simulink model "robotarm_individual"  (R2018b)
settings: Solver=FixedStepAuto  StartTime=0.0  StopTime=options.T_train-options.dt  RelTol=1e-3  AbsTol=1e-6
undefined symbols (not defined in the file or in its folder): options
libraries: neural x132, simulink x4
(part 2 of 6)

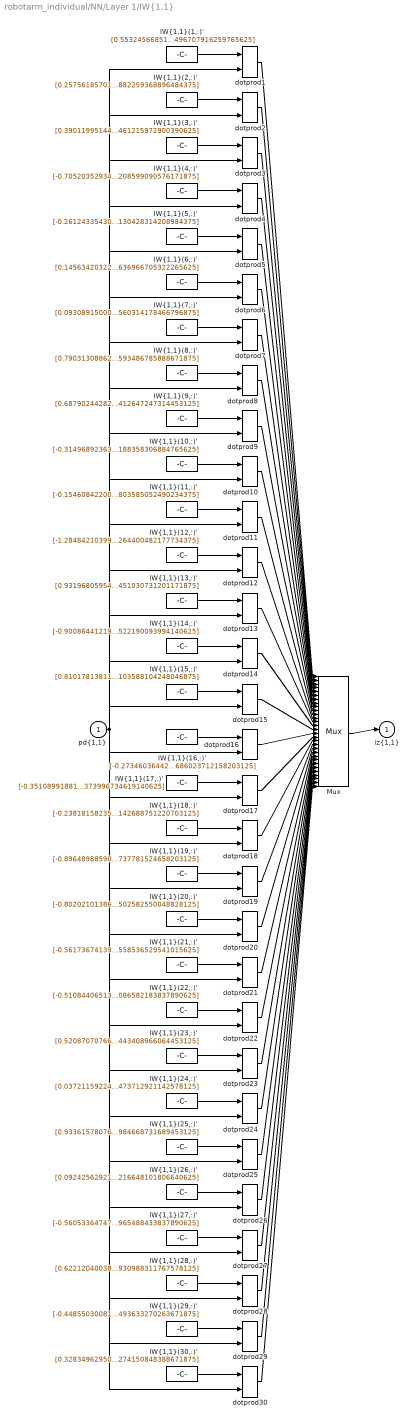
== system robotarm_individual/NN/Layer 1/IW{1,1} ==
  "pd{1,1}" : Inport  PortDimensions=10
      mask Display: e = 0.06;c1 = [120 230 180]/255;c2 = ([120 230 180]+0)/(256+128);c3 = ([120 230 180]+128)/(256+128);patch([0 1 1 0],[0 0 1 1],c1);patch([0 1 1 1-e 1-e 0+e],[0 0 1 1-e 0+e 0+e],c2);patch([0 0 1 1-e 0+e 0+e],[0 1 1 1-e 1-e 0+e],c3);plot([0 1 1 0 0],[0 0 1 1 0]);
  "IW{1,1}(1,:)'" : Constant  Value=[0.5532456685171613930407374937203712761402130126953125;-0.378274693650503757158531925597344525158405303955078125;0.56914966942954603457138773592305369675159454345703125;-0.50553199151917294074110031942836940288543701171875;0.658232888932551052363351118401624262332916259765625;-0.94884153385445257899988291683257557451725006103515625;0.473460329120412637404768929627607576549053192138671875;-0.343214399203028375229251878408831544220447540283203125;-0.86431174897959639480404803180135786533355712890625;0.589926606124411279097330407239496707916259765625]
      mask Display: e = 0.06;c1 = [120 150 230]/255;c2 = ([120 150 230]+0)/383;c3 = ([120 150 230]+128)/383;patch([0 1 1 0],[0 0 1 1],c1);patch([0 1 1 1-e 1-e 0+e],[0 0 1 1-e 0+e 0+e],c2);patch([0 0 1 1-e 0+e 0+e],[0 1 1 1-e 1-e 0+e],c3);plot([0 1 1 0 0],[0 0 1 1 0]);disp('Weights');
  "IW{1,1}(10,:)'" : Constant  Value=[-0.31496892363713457907437032190500758588314056396484375;0.08016139377854337999540490500294254161417484283447265625;-0.61410989189934184206975942288408987224102020263671875;0.83386729739820009132955647146445699036121368408203125;0.57799131071100695589137785646016709506511688232421875;-0.6262339995467105513426986362901516258716583251953125;-0.7518840900690875184153583177248947322368621826171875;-0.26218799647532831098573069539270363748073577880859375;0.8278812331514815436861454145400784909725189208984375;0.08425980137559320459761380561758414842188358306884765625]
      mask Display: e = 0.06;c1 = [120 150 230]/255;c2 = ([120 150 230]+0)/383;c3 = ([120 150 230]+128)/383;patch([0 1 1 0],[0 0 1 1],c1);patch([0 1 1 1-e 1-e 0+e],[0 0 1 1-e 0+e 0+e],c2);patch([0 0 1 1-e 0+e 0+e],[0 1 1 1-e 1-e 0+e],c3);plot([0 1 1 0 0],[0 0 1 1 0]);disp('Weights');
  "IW{1,1}(11,:)'" : Constant  Value=[-0.154608422005096890483599736398900859057903289794921875;0.68411476946963423184655539444065652787685394287109375;1.2591100033743873876090901831048540771007537841796875;0.1916528314192149640149409606237895786762237548828125;0.73897937867888419116724207924562506377696990966796875;-0.462187568499372092301058501107036136090755462646484375;-0.6040747226094336230772796625387854874134063720703125;0.36621315421464040174015508455340750515460968017578125;-0.372145694478708488617257899022661149501800537109375;0.78331781670854760957212192806764505803585052490234375]
      mask Display: e = 0.06;c1 = [120 150 230]/255;c2 = ([120 150 230]+0)/383;c3 = ([120 150 230]+128)/383;patch([0 1 1 0],[0 0 1 1],c1);patch([0 1 1 1-e 1-e 0+e],[0 0 1 1-e 0+e 0+e],c2);patch([0 0 1 1-e 0+e 0+e],[0 1 1 1-e 1-e 0+e],c3);plot([0 1 1 0 0],[0 0 1 1 0]);disp('Weights');
  "IW{1,1}(12,:)'" : Constant  Value=[-1.28484210399403142588425907888449728488922119140625;0.22635365405415874828776168214972130954265594482421875;0.1816503187597983959289393851577187888324260711669921875;-0.1064881354629866605510102317566634155809879302978515625;-1.0462119922659776083406768520944751799106597900390625;0.5159786559938523975432644874672405421733856201171875;-0.8176738284437050641173527765204198658466339111328125;0.55055084348684513173566301702521741390228271484375;0.7383955129630279667907188922981731593608856201171875;0.19266224517703045560068630948080681264400482177734375]
      mask Display: e = 0.06;c1 = [120 150 230]/255;c2 = ([120 150 230]+0)/383;c3 = ([120 150 230]+128)/383;patch([0 1 1 0],[0 0 1 1],c1);patch([0 1 1 1-e 1-e 0+e],[0 0 1 1-e 0+e 0+e],c2);patch([0 0 1 1-e 0+e 0+e],[0 1 1 1-e 1-e 0+e],c3);plot([0 1 1 0 0],[0 0 1 1 0]);disp('Weights');
  "IW{1,1}(13,:)'" : Constant  Value=[0.93196805954806338778695362634607590734958648681640625;-0.3434030090779085497842970653437077999114990234375;0.26082198307258275260522850658162496984004974365234375;0.96324277405090830139755553318536840379238128662109375;-0.0628666554734025606610003933383268304169178009033203125;0.1961376834922242962111482711407006718218326568603515625;0.426206572939244632269861767781549133360385894775390625;-0.09830317045506797857257197392755188047885894775390625;-0.56255042861082971139552455497323535382747650146484375;-0.9320516091341672915149274558643810451030731201171875]
      mask Display: e = 0.06;c1 = [120 150 230]/255;c2 = ([120 150 230]+0)/383;c3 = ([120 150 230]+128)/383;patch([0 1 1 0],[0 0 1 1],c1);patch([0 1 1 1-e 1-e 0+e],[0 0 1 1-e 0+e 0+e],c2);patch([0 0 1 1-e 0+e 0+e],[0 1 1 1-e 1-e 0+e],c3);plot([0 1 1 0 0],[0 0 1 1 0]);disp('Weights');
  "IW{1,1}(14,:)'" : Constant  Value=[-0.9008644121983826469346468002186156809329986572265625;0.313446134367460327307952638875576667487621307373046875;0.96742102718049050036341895975056104362010955810546875;0.60793812066105668012738760808133520185947418212890625;-0.66596089840168570805900571940583176910877227783203125;0.184208381037875235097800441508297808468341827392578125;1.04809193563155833572864139568991959095001220703125;0.1271048703670402957310869851426105014979839324951171875;0.162963867020818276021287829280481673777103424072265625;0.14456201261527967805164962555863894522190093994140625]
      mask Display: e = 0.06;c1 = [120 150 230]/255;c2 = ([120 150 230]+0)/383;c3 = ([120 150 230]+128)/383;patch([0 1 1 0],[0 0 1 1],c1);patch([0 1 1 1-e 1-e 0+e],[0 0 1 1-e 0+e 0+e],c2);patch([0 0 1 1-e 0+e 0+e],[0 1 1 1-e 1-e 0+e],c3);plot([0 1 1 0 0],[0 0 1 1 0]);disp('Weights');
  "IW{1,1}(15,:)'" : Constant  Value=[0.81017813811836136839161781608709134161472320556640625;-0.195009913062815176676423334356513805687427520751953125;0.932578705573031907505310300621204078197479248046875;-0.608942526772529912904019511188380420207977294921875;0.288607547931308439093101014805142767727375030517578125;0.410832973134562184913676219366607256233692169189453125;-0.5702079370302370886491871715406887233257293701171875;-0.834083175635048856833009267575107514858245849609375;-0.369136183700158937437407757897744886577129364013671875;-0.1105305058924390404495596840206417255103588104248046875]
      mask Display: e = 0.06;c1 = [120 150 230]/255;c2 = ([120 150 230]+0)/383;c3 = ([120 150 230]+128)/383;patch([0 1 1 0],[0 0 1 1],c1);patch([0 1 1 1-e 1-e 0+e],[0 0 1 1-e 0+e 0+e],c2);patch([0 0 1 1-e 0+e 0+e],[0 1 1 1-e 1-e 0+e],c3);plot([0 1 1 0 0],[0 0 1 1 0]);disp('Weights');
  "IW{1,1}(16,:)'" : Constant  Value=[-0.2734603644283737367004505358636379241943359375;-0.204328889329515150929950095815001986920833587646484375;0.59110685339935731263949492131359875202178955078125;-0.88973267111763887360353919575572945177555084228515625;-0.22325827977047263406262800344848074018955230712890625;-0.81981060084553381006600147884455509483814239501953125;0.310406978672233380134315439136116765439510345458984375;0.325731004946167301827841811245889402925968170166015625;-0.716110955615486322045626366161741316318511962890625;1.0571576827206012882953700682264752686023712158203125]
      mask Display: e = 0.06;c1 = [120 150 230]/255;c2 = ([120 150 230]+0)/383;c3 = ([120 150 230]+128)/383;patch([0 1 1 0],[0 0 1 1],c1);patch([0 1 1 1-e 1-e 0+e],[0 0 1 1-e 0+e 0+e],c2);patch([0 0 1 1-e 0+e 0+e],[0 1 1 1-e 1-e 0+e],c3);plot([0 1 1 0 0],[0 0 1 1 0]);disp('Weights');
  "IW{1,1}(17,:)'" : Constant  Value=[-0.351089918816565649262173565148259513080120086669921875;-0.5795299568452569882737179796095006167888641357421875;0.39367642982406392260230632018647156655788421630859375;-0.804876069961220963477899204008281230926513671875;-0.73883915685776513360139006181270815432071685791015625;0.7104609696887447256585801369510591030120849609375;-0.366867000264476550430714496542350389063358306884765625;0.2285119414857186281864187549217604100704193115234375;1.0456721991181769926271272197482176125049591064453125;0.2068165982501783961566843572654761373996734619140625]
      mask Display: e = 0.06;c1 = [120 150 230]/255;c2 = ([120 150 230]+0)/383;c3 = ([120 150 230]+128)/383;patch([0 1 1 0],[0 0 1 1],c1);patch([0 1 1 1-e 1-e 0+e],[0 0 1 1-e 0+e 0+e],c2);patch([0 0 1 1-e 0+e 0+e],[0 1 1 1-e 1-e 0+e],c3);plot([0 1 1 0 0],[0 0 1 1 0]);disp('Weights');
  "IW{1,1}(18,:)'" : Constant  Value=[-0.238181582357035959152113946402096189558506011962890625;-0.177534213017443043280962911012466065585613250732421875;0.74114288123727778412330735591240227222442626953125;-0.84890092028881902752601718020741827785968780517578125;0.51378812759981051794255790809984318912029266357421875;-0.4920295147625586285045073964283801615238189697265625;0.69652673017625144069597808993421494960784912109375;-0.2376268384348554085772065036508138291537761688232421875;0.8349156966200592666638158334535546600818634033203125;0.7017467499347926906949624026310630142688751220703125]
      mask Display: e = 0.06;c1 = [120 150 230]/255;c2 = ([120 150 230]+0)/383;c3 = ([120 150 230]+128)/383;patch([0 1 1 0],[0 0 1 1],c1);patch([0 1 1 1-e 1-e 0+e],[0 0 1 1-e 0+e 0+e],c2);patch([0 0 1 1-e 0+e 0+e],[0 1 1 1-e 1-e 0+e],c3);plot([0 1 1 0 0],[0 0 1 1 0]);disp('Weights');
  "IW{1,1}(19,:)'" : Constant  Value=[-0.89648988590438849488606365412124432623386383056640625;0.953009881848540185700358051690272986888885498046875;0.46992564373209610995019147594575770199298858642578125;-0.815624321845426880628338039969094097614288330078125;-0.370068889543076984249836414164747111499309539794921875;0.92926211570609584811109016300179064273834228515625;0.6792184335481394885647432602127082645893096923828125;-0.7702972690098748298481723395525477826595306396484375;0.187059012078736153217306537044350989162921905517578125;0.1501479221338375691363609121253830380737781524658203125]
      mask Display: e = 0.06;c1 = [120 150 230]/255;c2 = ([120 150 230]+0)/383;c3 = ([120 150 230]+128)/383;patch([0 1 1 0],[0 0 1 1],c1);patch([0 1 1 1-e 1-e 0+e],[0 0 1 1-e 0+e 0+e],c2);patch([0 0 1 1-e 0+e 0+e],[0 1 1 1-e 1-e 0+e],c3);plot([0 1 1 0 0],[0 0 1 1 0]);disp('Weights');
  "IW{1,1}(2,:)'" : Constant  Value=[0.257561857013934580873382174104335717856884002685546875;0.315507521129730517106537490690243430435657501220703125;0.03762196937497865045774148029522621072828769683837890625;-0.7714471080685851855918144792667590081691741943359375;0.324346761042450359990851893599028699100017547607421875;-0.7457496132203826899598197996965609490871429443359375;-0.398630963677156724411787536155316047370433807373046875;0.93888442215373657528942885619471780955791473388671875;0.64481812267807325778079530209652148187160491943359375;-0.03603365136383095135297338629243313334882259368896484375]
      mask Display: e = 0.06;c1 = [120 150 230]/255;c2 = ([120 150 230]+0)/383;c3 = ([120 150 230]+128)/383;patch([0 1 1 0],[0 0 1 1],c1);patch([0 1 1 1-e 1-e 0+e],[0 0 1 1-e 0+e 0+e],c2);patch([0 0 1 1-e 0+e 0+e],[0 1 1 1-e 1-e 0+e],c3);plot([0 1 1 0 0],[0 0 1 1 0]);disp('Weights');
  "IW{1,1}(20,:)'" : Constant  Value=[-0.80202101386553448225669171733898110687732696533203125;0.472829205768773352946965360388276167213916778564453125;0.790046357705378898828030287404544651508331298828125;0.92992033246759842057826972450129687786102294921875;-0.65014146895353863708777453211951069533824920654296875;0.11164351098992154887046268640915513969957828521728515625;0.261275402834526049300478689474402926862239837646484375;0.81302547517060597126459242645069025456905364990234375;0.36757030503491339157307038476574234664440155029296875;0.3011348129074875590305282457848079502582550048828125]
      mask Display: e = 0.06;c1 = [120 150 230]/255;c2 = ([120 150 230]+0)/383;c3 = ([120 150 230]+128)/383;patch([0 1 1 0],[0 0 1 1],c1);patch([0 1 1 1-e 1-e 0+e],[0 0 1 1-e 0+e 0+e],c2);patch([0 0 1 1-e 0+e 0+e],[0 1 1 1-e 1-e 0+e],c3);plot([0 1 1 0 0],[0 0 1 1 0]);disp('Weights');
  "IW{1,1}(21,:)'" : Constant  Value=[-0.56173674139086127166109463360044173896312713623046875;0.354869957496290633347513221451663412153720855712890625;-1.1424875621448602469598654352012090384960174560546875;0.20090882903061235698061182120000012218952178955078125;0.3719733516899841330172193920589052140712738037109375;-1.1174011975907964799858973492518998682498931884765625;0.37789935694898713069989071300369687378406524658203125;0.60326043740739809795314840812352485954761505126953125;0.377296422109360596319760361438966356217861175537109375;0.40403445130624560110987886218936182558536529541015625]
      mask Display: e = 0.06;c1 = [120 150 230]/255;c2 = ([120 150 230]+0)/383;c3 = ([120 150 230]+128)/383;patch([0 1 1 0],[0 0 1 1],c1);patch([0 1 1 1-e 1-e 0+e],[0 0 1 1-e 0+e 0+e],c2);patch([0 0 1 1-e 0+e 0+e],[0 1 1 1-e 1-e 0+e],c3);plot([0 1 1 0 0],[0 0 1 1 0]);disp('Weights');
  "IW{1,1}(22,:)'" : Constant  Value=[-0.51084406513362434765213038190267980098724365234375;-1.25725588359468787302830605767667293548583984375;0.032184547720003571502633832324136164970695972442626953125;-0.7225047379605715747175054275430738925933837890625;-0.5541908720409722821642617418547160923480987548828125;-0.1702807057209873853320658554366673342883586883544921875;0.71210533973892797821036992900189943611621856689453125;-0.1946879934669942524561037089370074681937694549560546875;0.62838588359199520905207236864953301846981048583984375;0.61014758277710579026376080946647562086582183837890625]
      mask Display: e = 0.06;c1 = [120 150 230]/255;c2 = ([120 150 230]+0)/383;c3 = ([120 150 230]+128)/383;patch([0 1 1 0],[0 0 1 1],c1);patch([0 1 1 1-e 1-e 0+e],[0 0 1 1-e 0+e 0+e],c2);patch([0 0 1 1-e 0+e 0+e],[0 1 1 1-e 1-e 0+e],c3);plot([0 1 1 0 0],[0 0 1 1 0]);disp('Weights');
  "IW{1,1}(23,:)'" : Constant  Value=[0.52087070766897658469218868049210868775844573974609375;-0.88570740858587015953418131175567395985126495361328125;-0.692278499514767720057761835050769150257110595703125;-0.165795948461607112189852841765969060361385345458984375;0.195788623739832468029220535754575394093990325927734375;0.3116435358859932502895162542699836194515228271484375;-0.415208131653555689855039645408396609127521514892578125;0.759006776227668655820934873190708458423614501953125;0.87231344430146950941207251162268221378326416015625;-0.0262245848892488642167819534734007902443408966064453125]
      mask Display: e = 0.06;c1 = [120 150 230]/255;c2 = ([120 150 230]+0)/383;c3 = ([120 150 230]+128)/383;patch([0 1 1 0],[0 0 1 1],c1);patch([0 1 1 1-e 1-e 0+e],[0 0 1 1-e 0+e 0+e],c2);patch([0 0 1 1-e 0+e 0+e],[0 1 1 1-e 1-e 0+e],c3);plot([0 1 1 0 0],[0 0 1 1 0]);disp('Weights');
  "IW{1,1}(24,:)'" : Constant  Value=[0.03721159224728003145354904290798003785312175750732421875;0.66481384878017479866940675492514856159687042236328125;-0.1653863284656953425155734294094145298004150390625;-0.4267748664224650934073679309221915900707244873046875;0.6537409873937576332281196300755254924297332763671875;-0.85207649239718252776043527774163521826267242431640625;0.85195534827163077462586215915507636964321136474609375;0.224894524523264693893764842869131825864315032958984375;0.375598544619615004602763974617118947207927703857421875;0.6846611303987437668894244779949076473712921142578125]
      mask Display: e = 0.06;c1 = [120 150 230]/255;c2 = ([120 150 230]+0)/383;c3 = ([120 150 230]+128)/383;patch([0 1 1 0],[0 0 1 1],c1);patch([0 1 1 1-e 1-e 0+e],[0 0 1 1-e 0+e 0+e],c2);patch([0 0 1 1-e 0+e 0+e],[0 1 1 1-e 1-e 0+e],c3);plot([0 1 1 0 0],[0 0 1 1 0]);disp('Weights');
  "IW{1,1}(25,:)'" : Constant  Value=[0.93361578076801532422024365587276406586170196533203125;0.329795848960595383569938121581799350678920745849609375;0.98232022553798248321044184194761328399181365966796875;-0.63958837546047797584236604961915872991085052490234375;0.94638989721688793199660949539975263178348541259765625;-0.6318542932302460002347288536839187145233154296875;0.0726763736254970316164047972051776014268398284912109375;-0.192350135202458305538897320730029605329036712646484375;0.0696687254914067077837813712903880514204502105712890625;0.0027320178679048241765503490796618280000984668731689453125]
      mask Display: e = 0.06;c1 = [120 150 230]/255;c2 = ([120 150 230]+0)/383;c3 = ([120 150 230]+128)/383;patch([0 1 1 0],[0 0 1 1],c1);patch([0 1 1 1-e 1-e 0+e],[0 0 1 1-e 0+e 0+e],c2);patch([0 0 1 1-e 0+e 0+e],[0 1 1 1-e 1-e 0+e],c3);plot([0 1 1 0 0],[0 0 1 1 0]);disp('Weights');
  "IW{1,1}(26,:)'" : Constant  Value=[0.0924256292148482871962045237523852847516536712646484375;-0.0860402085796024007624538398886215873062610626220703125;-0.377364887088004474779978636433952488005161285400390625;0.43311168102743813346222623295034281909465789794921875;0.983680985257372686447752130334265530109405517578125;0.945586219052464205248043072060681879520416259765625;-0.6454941091038122191747561373631469905376434326171875;-0.7499173601788291509961936753825284540653228759765625;0.3386455222846438406492097783484496176242828369140625;0.615331504743782176092281588353216648101806640625]
      mask Display: e = 0.06;c1 = [120 150 230]/255;c2 = ([120 150 230]+0)/383;c3 = ([120 150 230]+128)/383;patch([0 1 1 0],[0 0 1 1],c1);patch([0 1 1 1-e 1-e 0+e],[0 0 1 1-e 0+e 0+e],c2);patch([0 0 1 1-e 0+e 0+e],[0 1 1 1-e 1-e 0+e],c3);plot([0 1 1 0 0],[0 0 1 1 0]);disp('Weights');
  "IW{1,1}(27,:)'" : Constant  Value=[-0.5605336474717741435114248815807513892650604248046875;0.125243830871333339249673599624657072126865386962890625;1.14561265912899301611105329357087612152099609375;-0.4571008181785198853930296536418609321117401123046875;-0.27601301344836437490215530488057993352413177490234375;-0.2349407378672499768779147188979550264775753021240234375;0.62875068213826879048866658195038326084613800048828125;-0.98975657597570265711084402937558479607105255126953125;0.4570175005948178270642756615416146814823150634765625;0.6407066266972132329016176299774087965488433837890625]
      mask Display: e = 0.06;c1 = [120 150 230]/255;c2 = ([120 150 230]+0)/383;c3 = ([120 150 230]+128)/383;patch([0 1 1 0],[0 0 1 1],c1);patch([0 1 1 1-e 1-e 0+e],[0 0 1 1-e 0+e 0+e],c2);patch([0 0 1 1-e 0+e 0+e],[0 1 1 1-e 1-e 0+e],c3);plot([0 1 1 0 0],[0 0 1 1 0]);disp('Weights');
  "IW{1,1}(28,:)'" : Constant  Value=[0.62212040038602756109042957177734933793544769287109375;0.8669301188606770569577975038555450737476348876953125;0.788054740701710887407216432620771229267120361328125;0.64276933219258747254087893452378921210765838623046875;0.72944734222669216361367716672248207032680511474609375;0.6005279142654724733318971630069427192211151123046875;0.200537044405808495550758152603521011769771575927734375;0.474992803094998305990515063967905007302761077880859375;0.496268281793958931924493072074255906045436859130859375;-0.5413147400191242741840369490091688930988311767578125]
      mask Display: e = 0.06;c1 = [120 150 230]/255;c2 = ([120 150 230]+0)/383;c3 = ([120 150 230]+128)/383;patch([0 1 1 0],[0 0 1 1],c1);patch([0 1 1 1-e 1-e 0+e],[0 0 1 1-e 0+e 0+e],c2);patch([0 0 1 1-e 0+e 0+e],[0 1 1 1-e 1-e 0+e],c3);plot([0 1 1 0 0],[0 0 1 1 0]);disp('Weights');
  "IW{1,1}(29,:)'" : Constant  Value=[-0.448550300817549818521712268193368799984455108642578125;-0.2482488006127028246083909834851510822772979736328125;0.2533073445166624804159027917194180190563201904296875;-0.320151565141956917504018065301352180540561676025390625;-0.88425341610981045281647539013647474348545074462890625;0.24752485161112425249285706740920431911945343017578125;0.48636079906597740052376366293174214661121368408203125;0.84634390675732962261434977335738949477672576904296875;1.03789161496564741327119918423704802989959716796875;0.340648925443448546968028267656336538493633270263671875]
      mask Display: e = 0.06;c1 = [120 150 230]/255;c2 = ([120 150 230]+0)/383;c3 = ([120 150 230]+128)/383;patch([0 1 1 0],[0 0 1 1],c1);patch([0 1 1 1-e 1-e 0+e],[0 0 1 1-e 0+e 0+e],c2);patch([0 0 1 1-e 0+e 0+e],[0 1 1 1-e 1-e 0+e],c3);plot([0 1 1 0 0],[0 0 1 1 0]);disp('Weights');
  "IW{1,1}(3,:)'" : Constant  Value=[0.390119951448223922785274453417514450848102569580078125;0.748248336132188995861724833957850933074951171875;0.2034283677852984639766731334020732901990413665771484375;-0.58859623155779006165033706565736792981624603271484375;0.1134010025293597789808330844607553444802761077880859375;0.55907125571372906502887190072215162217617034912109375;0.5502027282670578500756164430640637874603271484375;-0.239874419150351847473956468093092553317546844482421875;0.8293755821765620428465126678929664194583892822265625;0.87892502878535305743668004652136005461215972900390625]
      mask Display: e = 0.06;c1 = [120 150 230]/255;c2 = ([120 150 230]+0)/383;c3 = ([120 150 230]+128)/383;patch([0 1 1 0],[0 0 1 1],c1);patch([0 1 1 1-e 1-e 0+e],[0 0 1 1-e 0+e 0+e],c2);patch([0 0 1 1-e 0+e 0+e],[0 1 1 1-e 1-e 0+e],c3);plot([0 1 1 0 0],[0 0 1 1 0]);disp('Weights');
  "IW{1,1}(30,:)'" : Constant  Value=[0.328349629504091578002800133617711253464221954345703125;-0.089013603511047201255479421888594515621662139892578125;0.29770821160272753491682351523195393383502960205078125;-0.89231689052477058954337962859426625072956085205078125;0.4492994321785366285126883667544461786746978759765625;-0.286915745348466588726665804642834700644016265869140625;0.88259032398641512617842863619443960487842559814453125;0.66350267602453161241982115825521759688854217529296875;-1.0133375026937867513510127537301741540431976318359375;-0.3026494383095410523054624718497507274150848388671875]
      mask Display: e = 0.06;c1 = [120 150 230]/255;c2 = ([120 150 230]+0)/383;c3 = ([120 150 230]+128)/383;patch([0 1 1 0],[0 0 1 1],c1);patch([0 1 1 1-e 1-e 0+e],[0 0 1 1-e 0+e 0+e],c2);patch([0 0 1 1-e 0+e 0+e],[0 1 1 1-e 1-e 0+e],c3);plot([0 1 1 0 0],[0 0 1 1 0]);disp('Weights');
  "IW{1,1}(4,:)'" : Constant  Value=[-0.70520352934453145454796185731538571417331695556640625;0.97785636573569367779867889112210832536220550537109375;-0.54029459356279352366669854745850898325443267822265625;-0.2371490475780859696897096000611782073974609375;-0.231390273644627331162126893104868941009044647216796875;0.288129384605261440466250633107847534120082855224609375;-0.186124598479057878908093925929279066622257232666015625;1.1160673461742776080285466377972625195980072021484375;0.490038125966539339639638228618423454463481903076171875;-0.315568469712563526297088856154005043208599090576171875]
      mask Display: e = 0.06;c1 = [120 150 230]/255;c2 = ([120 150 230]+0)/383;c3 = ([120 150 230]+128)/383;patch([0 1 1 0],[0 0 1 1],c1);patch([0 1 1 1-e 1-e 0+e],[0 0 1 1-e 0+e 0+e],c2);patch([0 0 1 1-e 0+e 0+e],[0 1 1 1-e 1-e 0+e],c3);plot([0 1 1 0 0],[0 0 1 1 0]);disp('Weights');
  "IW{1,1}(5,:)'" : Constant  Value=[-0.26124335430800404989071239469922147691249847412109375;0.32833996679531141094088297904818318784236907958984375;0.8255302241017303810366456673364154994487762451171875;0.80820115404521442048491053355974145233631134033203125;-0.357153555141686618323859647716744802892208099365234375;0.80745430468268419854638295873883180320262908935546875;-0.64542124945351286857686545772594399750232696533203125;0.56731945280087281435754675840144045650959014892578125;-0.8756858872747714794826379147707484662532806396484375;0.249905637820908965718302852110355161130428314208984375]
      mask Display: e = 0.06;c1 = [120 150 230]/255;c2 = ([120 150 230]+0)/383;c3 = ([120 150 230]+128)/383;patch([0 1 1 0],[0 0 1 1],c1);patch([0 1 1 1-e 1-e 0+e],[0 0 1 1-e 0+e 0+e],c2);patch([0 0 1 1-e 0+e 0+e],[0 1 1 1-e 1-e 0+e],c3);plot([0 1 1 0 0],[0 0 1 1 0]);disp('Weights');
  "IW{1,1}(6,:)'" : Constant  Value=[0.1456342032284982102030568285044864751398563385009765625;-0.460727603081207470747671095523401163518428802490234375;-0.2258479301822603202420935986083350144326686859130859375;-0.78049322745974902826304742120555602014064788818359375;-0.89402972148087200832122789506684057414531707763671875;0.96706161912398880264873923806590028107166290283203125;0.386161319623996190930625971304834820330142974853515625;0.285792775919690045238752418299554847180843353271484375;0.62880533399242855008282049311674199998378753662109375;0.16598592865024619502634095624671317636966705322265625]
      mask Display: e = 0.06;c1 = [120 150 230]/255;c2 = ([120 150 230]+0)/383;c3 = ([120 150 230]+128)/383;patch([0 1 1 0],[0 0 1 1],c1);patch([0 1 1 1-e 1-e 0+e],[0 0 1 1-e 0+e 0+e],c2);patch([0 0 1 1-e 0+e 0+e],[0 1 1 1-e 1-e 0+e],c3);plot([0 1 1 0 0],[0 0 1 1 0]);disp('Weights');
  "IW{1,1}(7,:)'" : Constant  Value=[0.0930891500094429835687748209238634444773197174072265625;-0.1397776829503553364109080803245888091623783111572265625;0.6091946803487797712506335301441140472888946533203125;-1.0513037741331896501861820070189423859119415283203125;-0.70221623447851400090513607210596092045307159423828125;-0.0696211597186368880141316139997798018157482147216796875;0.458984575880157397165248767123557627201080322265625;0.06853883520745594759571162057909532450139522552490234375;0.62199072355808338041782690197578631341457366943359375;-0.83952628838943876843359248596243560314178466796875]
      mask Display: e = 0.06;c1 = [120 150 230]/255;c2 = ([120 150 230]+0)/383;c3 = ([120 150 230]+128)/383;patch([0 1 1 0],[0 0 1 1],c1);patch([0 1 1 1-e 1-e 0+e],[0 0 1 1-e 0+e 0+e],c2);patch([0 0 1 1-e 0+e 0+e],[0 1 1 1-e 1-e 0+e],c3);plot([0 1 1 0 0],[0 0 1 1 0]);disp('Weights');
  "IW{1,1}(8,:)'" : Constant  Value=[0.7903130886230638196821018937043845653533935546875;-0.274840621338468815704203507266356609761714935302734375;-0.77669847149456117119115106106619350612163543701171875;0.6059040370284785037569008636637590825557708740234375;0.28922404260300649259107785837841220200061798095703125;-0.568491146563335547625683830119669437408447265625;0.492537579466517938531211484587402082979679107666015625;-0.348470456622766822096792793672648258507251739501953125;-0.7619226875622431283119340150733478367328643798828125;0.81202090607104338015886924040387384593486785888671875]
      mask Display: e = 0.06;c1 = [120 150 230]/255;c2 = ([120 150 230]+0)/383;c3 = ([120 150 230]+128)/383;patch([0 1 1 0],[0 0 1 1],c1);patch([0 1 1 1-e 1-e 0+e],[0 0 1 1-e 0+e 0+e],c2);patch([0 0 1 1-e 0+e 0+e],[0 1 1 1-e 1-e 0+e],c3);plot([0 1 1 0 0],[0 0 1 1 0]);disp('Weights');
  "IW{1,1}(9,:)'" : Constant  Value=[0.68790244282667789565977045640465803444385528564453125;-0.485533722471365669637322071139351464807987213134765625;1.0487205639455827732575698973960243165493011474609375;-0.64919493588700216690767774707637727260589599609375;-0.77821082144330777641272334221866913139820098876953125;0.88577302753543885049936079667531885206699371337890625;0.340546797832400327532553774290136061608791351318359375;-0.8062440005943074528005354295601136982440948486328125;0.36436416871731547306723086876445449888706207275390625;0.0981178621665923789141317001849529333412647247314453125]
      mask Display: e = 0.06;c1 = [120 150 230]/255;c2 = ([120 150 230]+0)/383;c3 = ([120 150 230]+128)/383;patch([0 1 1 0],[0 0 1 1],c1);patch([0 1 1 1-e 1-e 0+e],[0 0 1 1-e 0+e 0+e],c2);patch([0 0 1 1-e 0+e 0+e],[0 1 1 1-e 1-e 0+e],c3);plot([0 1 1 0 0],[0 0 1 1 0]);disp('Weights');
  Mux : Mux  Inputs=30
      mask Display: e = 0.06;c1 = [120 150 230]/255;c2 = ([120 150 230]+0)/383;c3 = ([120 150 230]+128)/383;patch([0 1 1 0],[0 0 1 1],c1);patch([0 1 1 1-e 1-e 0+e],[0 0 1 1-e 0+e 0+e],c2);patch([0 0 1 1-e 0+e 0+e],[0 1 1 1-e 1-e 0+e],c3);plot([0 1 1 0 0],[0 0 1 1 0]);disp('Mux');
  dotprod{1..30} (30 alike) : neural/Weight Functions/dotprod
  "iz{1,1}" : Outport
      mask Display: e = 0.06;c1 = [120 230 180]/255;c2 = ([120 230 180]+0)/(256+128);c3 = ([120 230 180]+128)/(256+128);patch([0 1 1 0],[0 0 1 1],c1);patch([0 1 1 1-e 1-e 0+e],[0 0 1 1-e 0+e 0+e],c2);patch([0 0 1 1-e 0+e 0+e],[0 1 1 1-e 1-e 0+e],c3);plot([0 1 1 0 0],[0 0 1 1 0]);
  wires:
  "IW{1,1}(1,:)'"/1 -> dotprod1/1
  "pd{1,1}"/1 -> dotprod1/2, dotprod2/2, dotprod3/2, dotprod4/2, dotprod5/2, dotprod6/2, dotprod7/2, dotprod8/2, dotprod9/2, dotprod10/2, dotprod11/2, dotprod12/2, dotprod13/2, dotprod14/2, dotprod15/2, dotprod16/2, dotprod17/2, dotprod18/2, dotprod19/2, dotprod20/2, dotprod21/2, dotprod22/2, dotprod23/2, dotprod24/2, dotprod25/2, dotprod26/2, dotprod27/2, dotprod28/2, dotprod29/2, dotprod30/2
  dotprod1/1 -> Mux/1
  "IW{1,1}(2,:)'"/1 -> dotprod2/1
  dotprod2/1 -> Mux/2
  "IW{1,1}(3,:)'"/1 -> dotprod3/1
  dotprod3/1 -> Mux/3
  "IW{1,1}(4,:)'"/1 -> dotprod4/1
  dotprod4/1 -> Mux/4
  "IW{1,1}(5,:)'"/1 -> dotprod5/1
  dotprod5/1 -> Mux/5
  "IW{1,1}(6,:)'"/1 -> dotprod6/1
  dotprod6/1 -> Mux/6
  "IW{1,1}(7,:)'"/1 -> dotprod7/1
  dotprod7/1 -> Mux/7
  "IW{1,1}(8,:)'"/1 -> dotprod8/1
  dotprod8/1 -> Mux/8
  "IW{1,1}(9,:)'"/1 -> dotprod9/1
  dotprod9/1 -> Mux/9
  "IW{1,1}(10,:)'"/1 -> dotprod10/1
  dotprod10/1 -> Mux/10
  "IW{1,1}(11,:)'"/1 -> dotprod11/1
  dotprod11/1 -> Mux/11
  "IW{1,1}(12,:)'"/1 -> dotprod12/1
  dotprod12/1 -> Mux/12
  "IW{1,1}(13,:)'"/1 -> dotprod13/1
  dotprod13/1 -> Mux/13
  "IW{1,1}(14,:)'"/1 -> dotprod14/1
  dotprod14/1 -> Mux/14
  "IW{1,1}(15,:)'"/1 -> dotprod15/1
  dotprod15/1 -> Mux/15
  "IW{1,1}(16,:)'"/1 -> dotprod16/1
  dotprod16/1 -> Mux/16
  "IW{1,1}(17,:)'"/1 -> dotprod17/1
  dotprod17/1 -> Mux/17
  "IW{1,1}(18,:)'"/1 -> dotprod18/1
  dotprod18/1 -> Mux/18
  "IW{1,1}(19,:)'"/1 -> dotprod19/1
  dotprod19/1 -> Mux/19
  "IW{1,1}(20,:)'"/1 -> dotprod20/1
  dotprod20/1 -> Mux/20
  "IW{1,1}(21,:)'"/1 -> dotprod21/1
  dotprod21/1 -> Mux/21
  "IW{1,1}(22,:)'"/1 -> dotprod22/1
  dotprod22/1 -> Mux/22
  "IW{1,1}(23,:)'"/1 -> dotprod23/1
  dotprod23/1 -> Mux/23
  "IW{1,1}(24,:)'"/1 -> dotprod24/1
  dotprod24/1 -> Mux/24
  "IW{1,1}(25,:)'"/1 -> dotprod25/1
  dotprod25/1 -> Mux/25
  "IW{1,1}(26,:)'"/1 -> dotprod26/1
  dotprod26/1 -> Mux/26
  "IW{1,1}(27,:)'"/1 -> dotprod27/1
  dotprod27/1 -> Mux/27
  "IW{1,1}(28,:)'"/1 -> dotprod28/1
  dotprod28/1 -> Mux/28
  "IW{1,1}(29,:)'"/1 -> dotprod29/1
  dotprod29/1 -> Mux/29
  "IW{1,1}(30,:)'"/1 -> dotprod30/1
  dotprod30/1 -> Mux/30
  Mux/1 -> "iz{1,1}"/1

== system robotarm_individual/NN/Layer 2/Delays 1 ==
  "p{2}" : Inport  PortDimensions=30
      mask Display: e = 0.06;c1 = [120 230 180]/255;c2 = ([120 230 180]+0)/(256+128);c3 = ([120 230 180]+128)/(256+128);patch([0 1 1 0],[0 0 1 1],c1);patch([0 1 1 1-e 1-e 0+e],[0 0 1 1-e 0+e 0+e],c2);patch([0 0 1 1-e 0+e 0+e],[0 1 1 1-e 1-e 0+e],c3);plot([0 1 1 0 0],[0 0 1 1 0]);
  mux : Mux  Inputs=1
      mask Display: e = 0.06;c1 = [120 150 230]/255;c2 = ([120 150 230]+0)/383;c3 = ([120 150 230]+128)/383;patch([0 1 1 0],[0 0 1 1],c1);patch([0 1 1 1-e 1-e 0+e],[0 0 1 1-e 0+e 0+e],c2);patch([0 0 1 1-e 0+e 0+e],[0 1 1 1-e 1-e 0+e],c3);plot([0 1 1 0 0],[0 0 1 1 0]);disp('Mux')
  "pd{2,1}" : Outport
      mask Display: e = 0.06;c1 = [120 230 180]/255;c2 = ([120 230 180]+0)/(256+128);c3 = ([120 230 180]+128)/(256+128);patch([0 1 1 0],[0 0 1 1],c1);patch([0 1 1 1-e 1-e 0+e],[0 0 1 1-e 0+e 0+e],c2);patch([0 0 1 1-e 0+e 0+e],[0 1 1 1-e 1-e 0+e],c3);plot([0 1 1 0 0],[0 0 1 1 0]);
  wires:
  "p{2}"/1 -> mux/1
  mux/1 -> "pd{2,1}"/1
